simulink model "hyd_hyb_2_opt_cont_test_new_1_loc_rod_fin"  (Simulink 7.7)
settings: Solver=ode14x  StartTime=0  StopTime=560  FixedStep=0.01  MaxStep=.4  RelTol=1e-8
InitFcn:
  | const_3
values from neighbouring files (symbols this model uses):
  Af = 6.3    [brk_enrg.m]    (also in brk_enrg_1.m)
  BSFC_906_205 = [3.5684 4.3466 5.1668 6.0769 6.988 7.8992 8.8104 9.7336 10.8548 11.9809 13.1112 14.2571 ... (663 elements, 39x17)]    [BSFC_map_906_205.mat]
  Cd = 0.55    [brk_enrg.m]    (also in brk_enrg_1.m)
  den = 1.202    [brk_enrg.m]    (also in brk_enrg_1.m)
  fr = 0.01    [brk_enrg.m]    (also in brk_enrg_1.m)
undefined symbols (not defined in the file or in its folder): clutchRise, down_spd_2, down_spd_3, down_spd_4, down_spd_c, fuel_density, gearshift, I_wheel, Idle_spd_eng_906, M1_hydr, p_v_15, pmax_125, qv_125, Rw, sec_eng_sfc_map, T_max_906, T_min, TC_spd_ratio_max, torque_convertor, Twait, up_spd_1, up_spd_2, up_spd_3, up_spd_c, v_p_10, v_p_15, v_p_5
libraries: neural x327, fl_lib x43, nesl_utility x30, sdl_lib x14, simulink x4, simulink_need_slupdate x1
(part 10 of 10)

== system hyd_hyb_2_opt_cont_test_new_1_loc_rod_fin/controller1/optimized controller - pm1/net_loc_rod_3/Layer 3/Delays 1 ==
  "p{3}" : Inport  PortDimensions=50
      mask Display: e = 0.06;c1 = [120 230 180]/255;c2 = ([120 230 180]+0)/(256+128);c3 = ([120 230 180]+128)/(256+128);patch([0 1 1 0],[0 0 1 1],c1);patch([0 1 1 1-e 1-e 0+e],[0 0 1 1-e 0+e 0+e],c2);patch([0 0 1 1-e 0+e 0+e],[0 1 1 1-e 1-e 0+e],c3);plot([0 1 1 0 0],[0 0 1 1 0]);
  mux : Mux  Inputs=1
      mask Display: e = 0.06;c1 = [120 150 230]/255;c2 = ([120 150 230]+0)/383;c3 = ([120 150 230]+128)/383;patch([0 1 1 0],[0 0 1 1],c1);patch([0 1 1 1-e 1-e 0+e],[0 0 1 1-e 0+e 0+e],c2);patch([0 0 1 1-e 0+e 0+e],[0 1 1 1-e 1-e 0+e],c3);plot([0 1 1 0 0],[0 0 1 1 0]);disp('Mux')
  "pd{3,2}" : Outport
      mask Display: e = 0.06;c1 = [120 230 180]/255;c2 = ([120 230 180]+0)/(256+128);c3 = ([120 230 180]+128)/(256+128);patch([0 1 1 0],[0 0 1 1],c1);patch([0 1 1 1-e 1-e 0+e],[0 0 1 1-e 0+e 0+e],c2);patch([0 0 1 1-e 0+e 0+e],[0 1 1 1-e 1-e 0+e],c3);plot([0 1 1 0 0],[0 0 1 1 0]);
  wires:
  "p{3}"/1 -> mux/1
  mux/1 -> "pd{3,2}"/1

== system hyd_hyb_2_opt_cont_test_new_1_loc_rod_fin/controller1/optimized controller - pm1/net_loc_rod_3/Layer 3/LW{3,2} ==
  "ad{3,2}" : Inport  PortDimensions=50
      mask Display: e = 0.06;c1 = [120 230 180]/255;c2 = ([120 230 180]+0)/(256+128);c3 = ([120 230 180]+128)/(256+128);patch([0 1 1 0],[0 0 1 1],c1);patch([0 1 1 1-e 1-e 0+e],[0 0 1 1-e 0+e 0+e],c2);patch([0 0 1 1-e 0+e 0+e],[0 1 1 1-e 1-e 0+e],c3);plot([0 1 1 0 0],[0 0 1 1 0]);
  "IW{3,2}(1,:)'" : Constant  Value=[-0.053622316472408407;-0.84226494554242493;-0.011666555238415236;0.031159601043217352;-0.78268054928841213;-0.57151616164870489;1.4221727363549186;-0.10488946281125493;1.2411615794211213;0.43780555871349264;1.00493419279436;0.15002998915696672;1.3661578283373133;0.32486908955250487;-1.6329340060075963;-0.99013071211446091;-1.4892538432867246;0.26723088508392268;0.28734888528890729;0.58759079281789517;-0.1768652514762607;2.0048651876864887;0.56854832738280303;0.10563682831731072;-1.1861340597610985;-0.31187236193084056;-0.55652712678917171;-0.58570701720904939;-0.85769655120661814;-0.63504220012530976;-0.45945614747951691;-0.33497460021449971;0.44174526290521743;0.062041618499131916;0.68222669067813013;-1.0201721966018633;0.62059126174744772;0.95620224591382819;0.89174621526738795;-1.5292658096581986;-0.87351124103449762;0.1574652567038724;0.90406111130103139;0.70729979329683113;1.0917999447906963;0.85585506304082049;0.22171915966860506;0.075303211080594651;-0.96463296762836814;-1.4561106375539434]
      mask Display: e = 0.06;c1 = [120 150 230]/255;c2 = ([120 150 230]+0)/383;c3 = ([120 150 230]+128)/383;patch([0 1 1 0],[0 0 1 1],c1);patch([0 1 1 1-e 1-e 0+e],[0 0 1 1-e 0+e 0+e],c2);patch([0 0 1 1-e 0+e 0+e],[0 1 1 1-e 1-e 0+e],c3);plot([0 1 1 0 0],[0 0 1 1 0]);disp('weights');
  Mux : Mux  Inputs=1
      mask Display: e = 0.06;c1 = [120 150 230]/255;c2 = ([120 150 230]+0)/383;c3 = ([120 150 230]+128)/383;patch([0 1 1 0],[0 0 1 1],c1);patch([0 1 1 1-e 1-e 0+e],[0 0 1 1-e 0+e 0+e],c2);patch([0 0 1 1-e 0+e 0+e],[0 1 1 1-e 1-e 0+e],c3);plot([0 1 1 0 0],[0 0 1 1 0]);disp('Mux');
  dotprod1 : neural/Weight Functions/dotprod  SystemSampleTime=-1
  "lz{3,2}" : Outport
      mask Display: e = 0.06;c1 = [120 230 180]/255;c2 = ([120 230 180]+0)/(256+128);c3 = ([120 230 180]+128)/(256+128);patch([0 1 1 0],[0 0 1 1],c1);patch([0 1 1 1-e 1-e 0+e],[0 0 1 1-e 0+e 0+e],c2);patch([0 0 1 1-e 0+e 0+e],[0 1 1 1-e 1-e 0+e],c3);plot([0 1 1 0 0],[0 0 1 1 0]);
  wires:
  "IW{3,2}(1,:)'"/1 -> dotprod1/1
  "ad{3,2}"/1 -> dotprod1/2
  dotprod1/1 -> Mux/1
  Mux/1 -> "lz{3,2}"/1

== stateflow chart driver/Chart ==
  state transmission state control [group]
    state Drive
      during: s=1;
    state Neutral
      during: s=0;
    (default) -> Neutral
    Neutral -> Drive : [cyc> 0]
    Drive -> Neutral : after(1,sec)[cyc== 0]
  data: cyc input double; speed input double; s output double

== stateflow chart Transmission1/transmission control/Chart1 ==
  state fourth
    entry: gear = 4;
  state third
    entry: gear = 3;
  state second
    entry: gear = 2;
  state first
    entry: TC=1;
  state firstc
    entry: gear=1;
    entry: TC=0;
  second -> third [order 1] : after(Twait,tick)
      | [speed >= up_spd_2]
  first -> second [order 1] : after(Twait,tick)
      | [speed >= up_spd_1]
  third -> fourth [order 1] : after(Twait,tick)
      | [speed >= up_spd_3]
  firstc -> first : after(Twait,tick)
      | [speed >=up_spd_c]
  (default) -> firstc
  third -> second [order 2] : after(Twait,tick)
      | [speed < down_spd_3]
  fourth -> third : after(Twait,tick)
      | [speed < down_spd_4]
  first -> firstc [order 2] : after(Twait,tick)
      | [speed < down_spd_c]
  second -> first [order 2] : after(Twait,tick)
      | [speed < down_spd_2]
  data: speed input double; gear output double; TC output double; down_spd_4 parameter double; down_spd_2 parameter double; down_spd_3 parameter double; up_spd_1 parameter double; up_spd_2 parameter double; up_spd_3 parameter double; down_spd_c parameter double; up_spd_c parameter double; Twait parameter double

== matlab function controller1/MATLAB Function ==
  data: T_pm_1 input double; T_pm output double; T_eng output double; T_brk input double; T_dem input double; delta_p input double; T_mech_brk output double; T_eng_1 input double
function [T_pm,T_eng,T_mech_brk] = fcn(T_pm_1,T_brk,T_dem,delta_p,T_eng_1)
if abs(T_dem)>0
    if T_brk<0
        T_eng=0;T_pm=T_pm_1;
        if delta_p>=325
            T_pm=0;
        end
        T_mech_brk=min(0,T_brk-T_pm);
    else    
        T_mech_brk=0;
        T_pm=min(T_pm_1,(delta_p*650/325));
        if delta_p<=140
            T_pm=0;
        end
%         T_eng=max(0,T_dem-T_pm);
        T_eng=min(1100,T_eng_1);
        if T_eng<100
            T_eng=0;
            T_pm=T_dem;
        end
    end
else
    T_pm=0;T_eng=0;T_mech_brk=0;
end
end

== stateflow chart hydraulic transmission/PM_hydraulic_machine /qv - pmax evaluation/Chart ==
  state state1
    during: u1=1;
  state state2
    during: u1=0;
  (default) -> state1
  state1 -> state2 : [soc <= soc_min]
  state2 -> state1 : [soc > 50]
  data: soc input double; soc_min input double; u1 output double
